simulink model "AHRS_Android"  (R2022b)
settings: Solver=FixedStepAuto  StartTime=0.0  StopTime=inf  FixedStep=Ts  RelTol=1e-3
InitFcn:
  | Ts = 0.02
values from neighbouring files (symbols this model uses):
  Zt = [phi_ ... (first row only)    [AHRS_testdata.m]
undefined symbols (not defined in the file or in its folder): article_one, eulerdata, Mag_data, test
libraries: androiduilib x4, androidsensorlib x3, simulink_extras x2
settings Model: Creator=LENOVO  LastModifiedBy=LENOVO
settings OptimizationCC: EnhancedBackFolding=on  PassReuseOutputArgsAs=Individual arguments  ZeroExternalMemoryAtStartup=off  ZeroInternalMemoryAtStartup=off  MaxStackSize=64  OptimizeBlockOrder=speed  DifferentSizesBufferReuse=on  OptimizationCustomize=off  EfficientTunableParamExpr=on
settings DebuggingCC: ParameterPrecisionLossMsg=none  ParameterTunabilityLossMsg=error
settings HardwareCC: ProdBitPerLong=64  ProdLargestAtomicInteger=LongLong  ProdLargestAtomicFloat=Double  ProdLongLongMode=on  ProdHWDeviceType=ARM Compatible->ARM 64-bit (LP64)
settings SFSimCC: MATLABDynamicMemAlloc=off
settings RTWCC: Description=Embedded Coder  SystemTargetFile=ert.tlc  HardwareBoard=Android Device (64bit)  TLCOptions="-aInlineSetEventsForThisBaseRateFcn=TLC_FALSE -aSuppressMultiTaskScheduler=TLC_FALSE  -aRateBasedStepFcn=0"  TemplateMakefile=ert_default_tmf  RTWVerbose=off  Toolchain=Android SDK/NDK Tools
settings CodeAppCC: ForceParamTrailComments=on  IgnoreCustomStorageClasses=off  OperatorAnnotations=on  SimulinkDataObjDesc=on  SFDataObjDesc=on  InsertBlockDesc=on
settings ERTTargetCC: SupportVariableSizeSignals=on

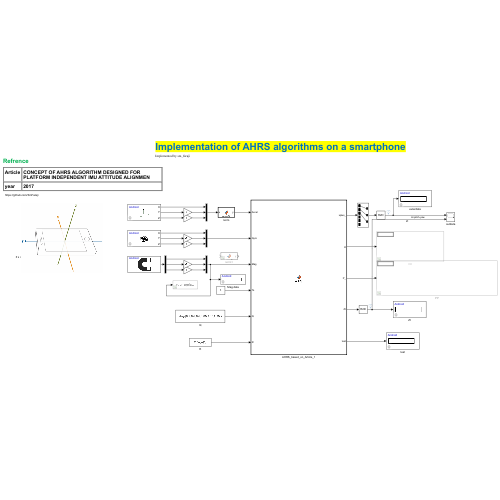
[thumbnail: Simulink's stored preview of the top-level diagram]
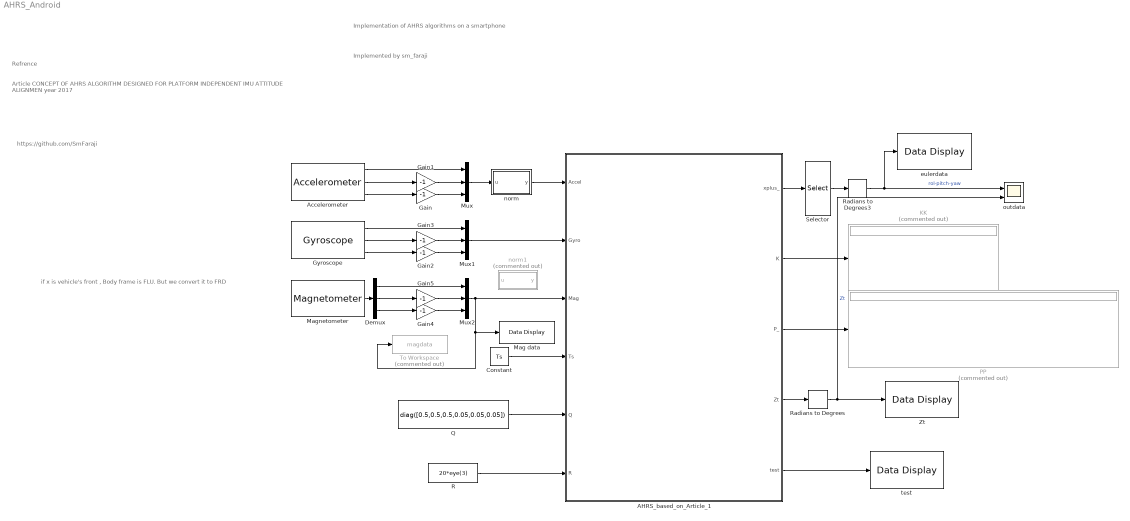
== system AHRS_Android ==
  note: https://github.com/SmFaraji
  note: if x is vehicle's front , Body frame is FLU. But we convert it to FRD
  note: Implemented by sm_faraji
  note: Implementation of AHRS algorithms on a smartphone
  note: Refrence
  note: Article
      | CONCEPT OF AHRS ALGORITHM DESIGNED FOR PLATFORM INDEPENDENT IMU ATTITUDE ALIGNMEN
      |
      | year
      | 2017
  AHRS_based_on_Article_1 : MATLAB Function  TreatAsAtomicUnit=on
  Accelerometer : androidsensorlib/Accelerometer  OutputVector=off  SampleTime=Ts  BlockPlatform=Android
  Constant : Constant  Value=Ts
  Demux : Demux  Outputs=3
  Gain{,1..5} (6 alike) : Gain  Gain=-1
  Gyroscope : androidsensorlib/Gyroscope  OutputVector=off  SampleTime=Ts  BlockPlatform=Android
  KK : Display  Commented=on
  Mag data : androiduilib/Data Display  DataDisplayId=article_one/Mag_data  Format=Float  Precision=6  SimulateUsing=Code generation  blockPlatform=Android
  Magnetometer : androidsensorlib/Magnetometer  SampleTime=Ts
  Mux : Mux  Inputs=3
  Mux1 : Mux  Inputs=3
  Mux2 : Mux  Inputs=3
  PP : Display  Commented=on
  Q : Constant  Value=diag([0.5,0.5,0.5,0.05,0.05,0.05])
  R : Constant  Value=20*eye(3)
  Radians to Degrees : simulink_extras/Transformations/Radians to Degrees
  Radians to Degrees3 : simulink_extras/Transformations/Radians to Degrees
  Selector : Selector  InputPortWidth=6  IndexOptions=Index vector (dialog)  Indices=[1:3]  OutputSizes=1
  To Workspace : ToWorkspace  Commented=on  VariableName=magdata  SampleTime=Ts
  Zt : androiduilib/Data Display  DataDisplayId=article_one/Zt  Format=Float  Precision=6  SimulateUsing=Code generation  blockPlatform=Android
  eulerdata : androiduilib/Data Display  DataDisplayId=article_one/eulerdata  Format=Float  Precision=6  SimulateUsing=Code generation  blockPlatform=Android
  norm : MATLAB Function  TreatAsAtomicUnit=on
  norm1 : MATLAB Function  Commented=on  TreatAsAtomicUnit=on
  outdata : Scope  NumInputPorts=2
  test : androiduilib/Data Display  DataDisplayId=article_one/test  Format=Float  Precision=6  SimulateUsing=Code generation  blockPlatform=Android
  wires:
  Accelerometer/3 -> Gain/1
  Accelerometer/2 -> Gain1/1
  Gyroscope/2 -> Gain3/1
  Gyroscope/3 -> Gain2/1
  Demux/2 -> Gain5/1
  Demux/3 -> Gain4/1
  Magnetometer/1 -> Demux/1
  Gain1/1 -> Mux/2
  Gain/1 -> Mux/3
  Accelerometer/1 -> Mux/1
  Gain3/1 -> Mux1/2
  Gain2/1 -> Mux1/3
  Gyroscope/1 -> Mux1/1
  Gain4/1 -> Mux2/3
  Gain5/1 -> Mux2/2
  Demux/1 -> Mux2/1
  Mux/1 -> norm/1(u)
  Constant/1 -> AHRS_based_on_Article_1/4(Ts)
  norm/1(y) -> AHRS_based_on_Article_1/1(Accel)
  Mux1/1 -> AHRS_based_on_Article_1/2(Gyro)
  AHRS_based_on_Article_1/1(xplus_) -> Selector/1
  AHRS_based_on_Article_1/3(P_) -> PP/1
  AHRS_based_on_Article_1/2(K) -> KK/1
  AHRS_based_on_Article_1/4(Zt) -> Radians to Degrees/1
  Radians to Degrees/1 -> outdata/2, Zt/1  "Zt"
  Selector/1 -> Radians to Degrees3/1
  Mux2/1 -> AHRS_based_on_Article_1/3(Mag), Mag data/1, To Workspace/1
  Q/1 -> AHRS_based_on_Article_1/5(Q)
  R/1 -> AHRS_based_on_Article_1/6(R)
  Radians to Degrees3/1 -> outdata/1, eulerdata/1  "rol-pitch-yaw"
  AHRS_based_on_Article_1/5(test) -> test/1

== matlab function AHRS_Android/norm ==
  data: u input; y output
function y = normV(u)
y = normalize(u,'norm');

== matlab function AHRS_Android/AHRS_based_on_Article_1 ==
  data: Accel input; xplus_ output; Gyro input; Mag input; Ts input; K output; P_ output; Zt output; Q input; R input; test output
function [xplus_,K,P_,Zt,test] = AHRS(Accel,Gyro,Mag,Ts,Q,R)



A = [1, 0, 0, -Ts,   0,  0;
     0, 1, 0,   0, -Ts,  0;
     0, 0, 1,   0,   0,-Ts;
     0, 0, 0,   1,   0,  0;
     0, 0, 0,   0,   1,  0;
     0, 0, 0,   0,   0,  1];
B = [Ts, 0, 0;
     0, Ts, 0;
     0,  0,Ts;
     0,  0, 0;
     0,  0, 0;
     0,  0, 0];
C = [1, 0, 0, 0, 0, 0;
     0, 1, 0, 0, 0, 0;
     0, 0, 1, 0, 0, 0];

                    
persistent P;
if isempty(P);P = Q; 
else 
    P = A*P*A' + Q;
end
P_=P;

S = C*P*C' + R; % Estimate error 
K = (P_*C')/S; % Kalman gain

%% meas
phi_ = -atan(Accel(2)/sqrt(Accel(1)^2+Accel(3)^2));
theta_ = atan(Accel(1)/sqrt(Accel(2)^2+Accel(3)^2));
Zt = [phi_;
      theta_;
      atan2(Mag(3) * sin(phi_) - Mag(2) * cos(phi_), Mag(1) * cos(theta_) + Mag(2) * sin(theta_) * sin(phi_) + Mag(3) * sin(theta_) * cos(phi_))  ];% atan2(-Mag(2),Mag(1))
test = [Mag(3) * sin(phi_) - Mag(2) * cos(phi_), Mag(1) * cos(theta_) + Mag(2) * sin(theta_) * sin(phi_) + Mag(3) * sin(theta_) * cos(phi_)];
persistent xplus
if isempty(xplus); xplus = [Zt;0;0;0];
else
x_ = A*xplus+B*(Gyro);
innov = Zt - C*x_ ;
xplus = x_ + K*innov;
end
xplus_ = xplus;

% Update the error covariance 

P_ = (eye(6) - K*C)*P_;
P = P_;

return

== matlab function AHRS_Android/norm1 ==
  data: u input; y output
function y = normV(u)
y = normalize(u,'norm');
